simulink model "PIDForCVCharging"  (R2018a)
settings: Solver=VariableStepAuto  StartTime=0.0  StopTime=30  RelTol=1e-3
values from neighbouring files (symbols this model uses):
  highVoltLimit = batteryParam.chargedVolt(cellID)    [script_initializeVariables_190821.m]
undefined symbols (not defined in the file or in its folder): re, rset
libraries: simulink x1
settings Model: Creator=100520035  LastModifiedBy=100520035

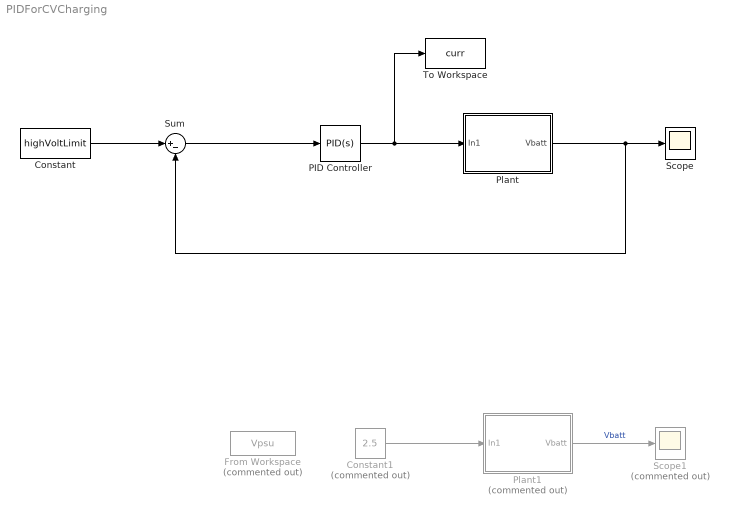
== system PIDForCVCharging ==
  Constant : Constant  Value=highVoltLimit
  Constant1 : Constant  Commented=on  Value=2.5
  From Workspace : FromWorkspace  Commented=on  VariableName=Vpsu  SampleTime=0
  PID Controller : simulink/Continuous/PID Controller  Controller=PID  TimeDomain=Continuous-time  SampleTime=-1  IntegratorMethod=Forward Euler  FilterMethod=Forward Euler  Form=Parallel  UseFilter=on  ControllerParametersSource=internal  P=0  I=6.94444444444444  D=0  N=100  InitialConditionSource=internal  InitialConditionForIntegrator=0  InitialConditionForFilter=0  ExternalReset=none  LimitOutput=off  UpperSaturationLimit=inf  LowerSaturationLimit=-inf  LinearizeAsGain=on  AntiWindupMode=none  Kb=1  TrackingMode=off  Kt=1  PParamMin=[]  PParamMax=[]  IParamMin=[]  IParamMax=[]  DParamMin=[]  DParamMax=[]  NParamMin=[]  NParamMax=[]  KbParamMin=[]  KbParamMax=[]  KtParamMin=[]  KtParamMax=[]  POutMin=[]  POutMax=[]  IOutMin=[]  IOutMax=[]  DOutMin=[]  DOutMax=[]  NOutMin=[]  NOutMax=[]  KbOutMin=[]  KbOutMax=[]  KtOutMin=[]  KtOutMax=[]  IntegratorOutMin=[]  IntegratorOutMax=[]  FilterOutMin=[]  FilterOutMax=[]  SumOutMin=[]  SumOutMax=[]  SumI1OutMin=[]  SumI1OutMax=[]  SumI2OutMin=[]  SumI2OutMax=[]  SumI3OutMin=[]  SumI3OutMax=[]  SumDOutMin=[]  SumDOutMax=[]  SaturationOutMin=[]  SaturationOutMax=[]  IntegratorContinuousStateAttributes=''  IntegratorStateMustResolveToSignalObject=off  IntegratorRTWStateStorageClass=Auto  FilterContinuousStateAttributes=''  FilterStateMustResolveToSignalObject=off  FilterRTWStateStorageClass=Auto  DifferentiatorICPrevScaledInput=0  DifferentiatorOutMin=[]  DifferentiatorOutMax=[]  FilterDiffOutCoefMin=[]  FilterDiffOutCoefMax=[]  SumDenOutMin=[]  SumDenOutMax=[]  SumNumOutMin=[]  SumNumOutMax=[]  ReciprocalOutMin=[]  ReciprocalOutMax=[]  DivideOutMin=[]  DivideOutMax=[]  TunerSelectOption=Transfer Function Based (PID Tuner App)
  Plant : Subsystem
  Plant1 : Subsystem  Commented=on
  Scope : Scope
  Scope1 : Scope  Commented=on
  Sum : Sum  Inputs=|+-
  To Workspace : ToWorkspace  VariableName=curr  SaveFormat=Timeseries  SampleTime=-1
  wires:
  Sum/1 -> PID Controller/1
  PID Controller/1 -> To Workspace/1, Plant/1(In1)
  Constant/1 -> Sum/1
  Plant1/1(Vbatt) -> Scope1/1  "Vbatt"
  Constant1/1 -> Plant1/1(In1)
  Plant/1(Vbatt) -> Sum/2, Scope/1

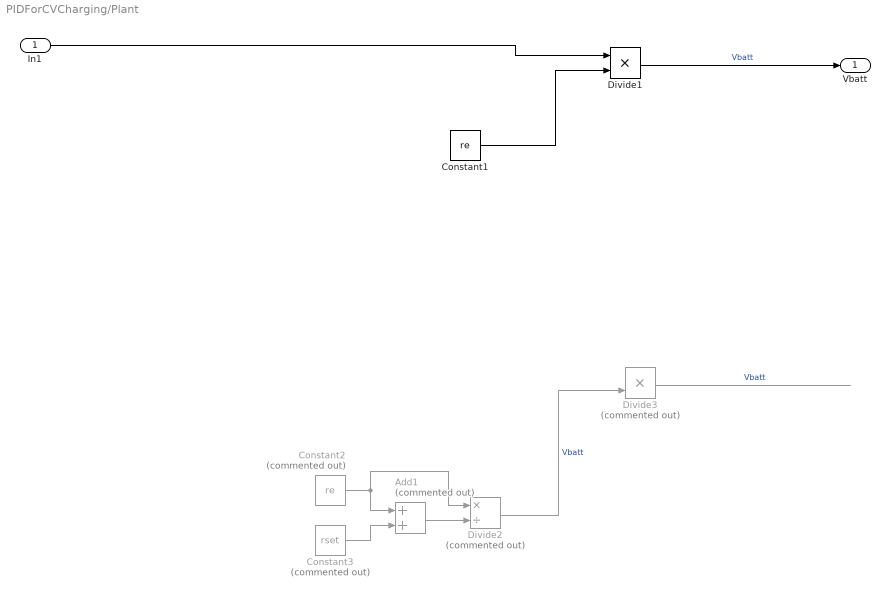
== system PIDForCVCharging/Plant ==
  In1 : Inport
  Add1 : Sum  Commented=on
  Constant1 : Constant  Value=re  OutDataTypeStr=double
  Constant2 : Constant  Commented=on  Value=re  OutDataTypeStr=double
  Constant3 : Constant  Commented=on  Value=rset
  Divide1 : Product
  Divide2 : Product  Commented=on  Inputs=*/
  Divide3 : Product  Commented=on
  Vbatt : Outport
  wires:
  In1/1 -> Divide1/1
  Divide1/1 -> Vbatt/1  "Vbatt"
  Divide3/1 -> ?  "Vbatt"
  Divide2/1 -> Divide3/2  "Vbatt"
  Constant2/1 -> Divide2/1, Add1/1
  Constant3/1 -> Add1/2
  Add1/1 -> Divide2/2
  ? -> Divide3/1
  Constant1/1 -> Divide1/2

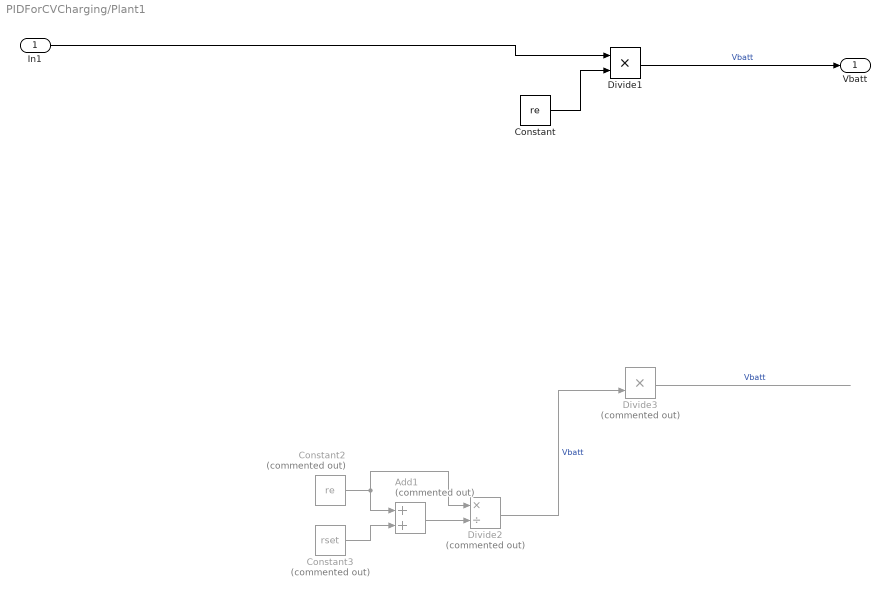
== system PIDForCVCharging/Plant1 ==
  In1 : Inport
  Add1 : Sum  Commented=on
  Constant : Constant  Value=re  OutDataTypeStr=double
  Constant2 : Constant  Commented=on  Value=re  OutDataTypeStr=double
  Constant3 : Constant  Commented=on  Value=rset
  Divide1 : Product
  Divide2 : Product  Commented=on  Inputs=*/
  Divide3 : Product  Commented=on
  Vbatt : Outport
  wires:
  Constant/1 -> Divide1/2
  ? -> Divide3/1
  Add1/1 -> Divide2/2
  Constant3/1 -> Add1/2
  Constant2/1 -> Add1/1, Divide2/1
  Divide2/1 -> Divide3/2  "Vbatt"
  Divide3/1 -> ?  "Vbatt"
  Divide1/1 -> Vbatt/1  "Vbatt"
  In1/1 -> Divide1/1
